simulink model "First_simulink"  (R2020a)
settings: Solver=VariableStepAuto  StartTime=0.0  StopTime=10.0  RelTol=1e-3
settings Model: Creator=User  LastModifiedBy=User

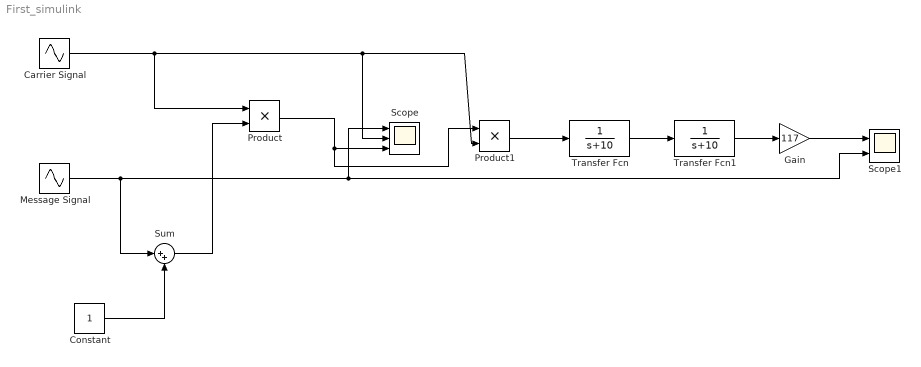
== system First_simulink ==
  Carrier Signal : Sin  Frequency=2*pi*25  SampleTime=1/5000
  Constant : Constant
  Gain : Gain  Gain=117
  Message Signal : Sin  Frequency=2*pi  SampleTime=1/5000
  Product : Product
  Product1 : Product
  Scope : Scope  NumInputPorts=3
  Scope1 : Scope  NumInputPorts=2
  Sum : Sum  Inputs=|++
  Transfer Fcn : TransferFcn  Denominator=[1 10]
  Transfer Fcn1 : TransferFcn  Denominator=[1 10]
  wires:
  Message Signal/1 -> Scope1/2, Scope/1, Sum/1
  Constant/1 -> Sum/2
  Sum/1 -> Product/2
  Product/1 -> Product1/1, Scope/3
  Carrier Signal/1 -> Product/1, Product1/2, Scope/2
  Product1/1 -> Transfer Fcn/1
  Transfer Fcn/1 -> Transfer Fcn1/1
  Transfer Fcn1/1 -> Gain/1
  Gain/1 -> Scope1/1
